simulink library "roundToN"  (R2018b)
settings: Solver=VariableStepAuto  StartTime=0.0  StopTime=10.0  RelTol=1e-3
settings Model: Creator=mcobb  LastModifiedBy=mcobb

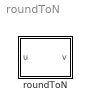
== system roundToN ==
  roundToN : Subsystem  mask{N=0}
      mask prompts: N "Number of Decimal Places"

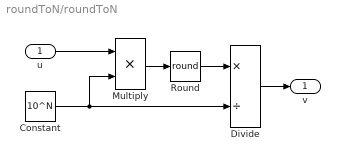
== system roundToN/roundToN ==
  u : Inport
  Constant : Constant  Value=10^N
  Divide : Product  Inputs=*/
  Multiply : Product
  Round : Rounding  Operator=round
  v : Outport
  wires:
  Round/1 -> Divide/1
  Divide/1 -> v/1
  Constant/1 -> Multiply/2, Divide/2
  Multiply/1 -> Round/1
  u/1 -> Multiply/1
